simulink model "OnOff"  (R2026a)
settings: Solver=FixedStepDiscrete  StopTime=0  EnableMultiTasking=on
settings Model: Creator=glenn gomes  LastModifiedBy=Nehir RT
settings DebuggingCC: UnderspecifiedInitializationDetection=Classic
settings HardwareCC: ProdHWDeviceType=32-bit Generic

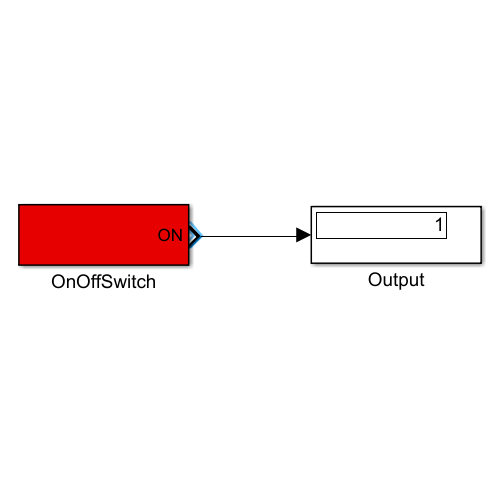
[thumbnail: Simulink's stored preview of the top-level diagram]
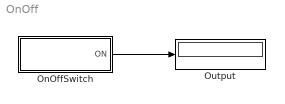
== system OnOff ==
  OnOffSwitch : Subsystem
      settings: OpenFcn=|
      | blockname1=[gcb '/ControlValue/'];
      | blockname2=[gcb '/'];
      | 
      | h1=get_param(blockname1,'handle');
      | h2=get_param(blockname2,'handle');
      | ONOFF=str2num(get_param(h1,'Value'));
      | 
      | if ONOFF== 1
      |     %Turn off
      |     set_param(h1,'Value','-1')
      |     set_param(h2,'BackgroundColor','blue')
      |     set_param([gcb '/ON'],'Name','OFF')
      | else
      |     %Turn on
      |     set_param(h1,'Value','1')
      |     set_param(h2,'BackgroundColor','red')
      |     set_param([gcb '/OFF'],'Name','ON')
      | end
  Output : Display
  wires:
  OnOffSwitch/1(ON) -> Output/1

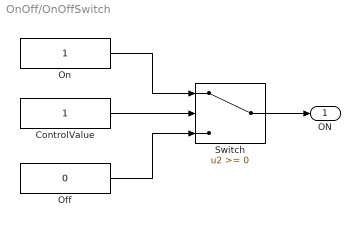
== system OnOff/OnOffSwitch ==
  ControlValue : Constant
  Off : Constant  Value=0
  On : Constant
  Switch : Switch  SaturateOnIntegerOverflow=off  InputSameDT=off
  ON : Outport
  wires:
  On/1 -> Switch/1
  Off/1 -> Switch/3
  ControlValue/1 -> Switch/2
  Switch/1 -> ON/1
